simulink model "Combined_Experiment_Jan23_2020a"  (R2020a)
settings: Solver=FixedStepAuto  StartTime=0.0  StopTime=tsim  FixedStep=baseRate  RelTol=1e-3  EnableMultiTasking=on
undefined symbols (not defined in the file): b0, b1, b_out, baseRate, CHASER_ABSOLUTE_POSITION, DiscIntNeverNeededParam, drop_states_ARM, drop_states_BLACK, drop_states_BLUE, drop_states_RED, F_Black_X_nominal, F_Black_Y_nominal, F_Blue_X_nominal, F_Blue_Y_nominal, F_red_X_nominal, F_red_Y_nominal, F_thrusters_BLACK, F_thrusters_BLUE, F_thrusters_RED, Gamma1_el, Gamma1_sh, Gamma1_wr, Gamma2_el, Gamma2_sh, Gamma2_wr, Gamma3_el, Gamma3_sh, Gamma3_wr, Gamma4_el, Gamma4_sh, Gamma4_wr, Gamma5_el, Gamma5_sh, Gamma5_wr, Gamma6_el, Gamma6_sh, Gamma6_wr, home_states_BLACK, home_states_BLUE, home_states_RED, init_states_BLACK, init_states_BLUE, init_states_RED, Kd_tb, Kd_tblue, Kd_tr, Kd_xb, Kd_xblue, Kd_xr, Kd_yb, Kd_yblue, Kd_yr, Kp_tb, Kp_tblue, Kp_tr, Kp_xb, Kp_xblue, Kp_xr, Kp_yb, Kp_yblue ... (+31)
libraries: dspstat3 x18, raspberrypiBasiclib x10, dspsigops x9, embdlinuxlib x8, MainLibrary x8, simulink x7, mspfiltlib x3, dsparch4 x3, etargetslib x1, sensehatlib x1
(part 2 of 11)

== system Combined_Experiment_Jan23_2020a/Manipulator Initialization ==
  Change BLACK Behavior : Subsystem  TreatAsAtomicUnit=on
  Change BLUE Behavior : Subsystem  TreatAsAtomicUnit=on
  Change RED Behavior : Subsystem  TreatAsAtomicUnit=on
  Data Store Read : DataStoreRead  DataStoreName=WhoAmI
  Is this a simulation? : Subsystem
  This IF block determines whether or not to run the BLACK sim/exp : If  NumInputs=2  IfExpression=u1 == 2 & u2 == 0  ShowElse=off
  This IF block determines whether or not to run the BLUE sim/exp : If  NumInputs=2  IfExpression=u1 == 3 & u2 == 0  ShowElse=off
  "This IF block determines whether or not to run the RED sim/exp " : If  NumInputs=2  IfExpression=u1 == 1 & u2 ==0  ShowElse=off
  wires:
  "This IF block determines whether or not to run the RED sim/exp "/1 -> Change RED Behavior/Action
  This IF block determines whether or not to run the BLACK sim/exp/1 -> Change BLACK Behavior/Action
  Is this a simulation?/1(isSim) -> This IF block determines whether or not to run the BLACK sim/exp/2, This IF block determines whether or not to run the BLUE sim/exp/2, "This IF block determines whether or not to run the RED sim/exp "/2
  Data Store Read/1 -> This IF block determines whether or not to run the BLUE sim/exp/1, This IF block determines whether or not to run the BLACK sim/exp/1, "This IF block determines whether or not to run the RED sim/exp "/1
  This IF block determines whether or not to run the BLUE sim/exp/1 -> Change BLUE Behavior/Action

== system Combined_Experiment_Jan23_2020a/Phase #0: Wait for Synchronization ==
  note: In this subsection, the "if" statements are used to determine two things: 1) whether or not a simulation is begin performed,
      | then 2) if an experiment is being performed, then which platform is the diagram compiled on. The "IdentifyPlatform" variable
      | is obtained from a text file location on each platform; each text file contains a unique identifier for each platform.
  Action Port : ActionPort  ActionPortLabel=if(u1 < u2)
  Change BLACK Behavior : Subsystem  TreatAsAtomicUnit=on
  Change BLUE Behavior : Subsystem  TreatAsAtomicUnit=on
  Change RED Behavior : Subsystem  TreatAsAtomicUnit=on
  Data Store Read : DataStoreRead  DataStoreName=WhoAmI
  Is this a simulation? : Subsystem
  This IF block determines whether or not to run the BLACK sim/exp : If  NumInputs=2  IfExpression=u1 == 2 | u2 == 1  ShowElse=off
  This IF block determines whether or not to run the BLUE sim/exp : If  NumInputs=2  IfExpression=u1 == 3 | u2 == 1  ShowElse=off
  "This IF block determines whether or not to run the RED sim/exp " : If  NumInputs=2  IfExpression=u1 == 1 | u2 == 1  ShowElse=off
  wires:
  Is this a simulation?/1(isSim) -> This IF block determines whether or not to run the BLACK sim/exp/2, This IF block determines whether or not to run the BLUE sim/exp/2, "This IF block determines whether or not to run the RED sim/exp "/2
  "This IF block determines whether or not to run the RED sim/exp "/1 -> Change RED Behavior/Action
  This IF block determines whether or not to run the BLACK sim/exp/1 -> Change BLACK Behavior/Action
  Data Store Read/1 -> This IF block determines whether or not to run the BLUE sim/exp/1, This IF block determines whether or not to run the BLACK sim/exp/1, "This IF block determines whether or not to run the RED sim/exp "/1
  This IF block determines whether or not to run the BLUE sim/exp/1 -> Change BLUE Behavior/Action

== system Combined_Experiment_Jan23_2020a/Phase #1: Start Floating  ==
  note: In this subsection, the "if" statements are used to determine two things: 1) whether or not a simulation is begin performed,
      | then 2) if an experiment is being performed, then which platform is the diagram compiled on. The "IdentifyPlatform" variable
      | is obtained from a text file location on each platform; each text file contains a unique identifier for each platform.
  Action Port : ActionPort  ActionPortLabel=elseif(u1 < u3)
  Change BLACK Behavior : Subsystem  TreatAsAtomicUnit=on
  Change BLUE Behavior : Subsystem  TreatAsAtomicUnit=on
  Change RED Behavior : Subsystem  TreatAsAtomicUnit=on
  Data Store Read : DataStoreRead  DataStoreName=WhoAmI
  Is this a simulation? : Subsystem
  This IF block determines whether or not to run the BLACK sim/exp : If  NumInputs=2  IfExpression=u1 == 2 | u2 == 1  ShowElse=off
  This IF block determines whether or not to run the BLUE sim/exp : If  NumInputs=2  IfExpression=u1 == 3 | u2 == 1  ShowElse=off
  "This IF block determines whether or not to run the RED sim/exp " : If  NumInputs=2  IfExpression=u1 == 1 | u2 == 1  ShowElse=off
  wires:
  "This IF block determines whether or not to run the RED sim/exp "/1 -> Change RED Behavior/Action
  This IF block determines whether or not to run the BLACK sim/exp/1 -> Change BLACK Behavior/Action
  Is this a simulation?/1(isSim) -> This IF block determines whether or not to run the BLUE sim/exp/2, This IF block determines whether or not to run the BLACK sim/exp/2, "This IF block determines whether or not to run the RED sim/exp "/2
  This IF block determines whether or not to run the BLUE sim/exp/1 -> Change BLUE Behavior/Action
  Data Store Read/1 -> This IF block determines whether or not to run the BLUE sim/exp/1, This IF block determines whether or not to run the BLACK sim/exp/1, "This IF block determines whether or not to run the RED sim/exp "/1

== system Combined_Experiment_Jan23_2020a/Phase #2: Move to Initial Position ==
  note: In this subsection, the "if" statements are used to determine two things: 1) whether or not a simulation is begin performed,
      | then 2) if an experiment is being performed, then which platform is the diagram compiled on. The "IdentifyPlatform" variable
      | is obtained from a text file location on each platform; each text file contains a unique identifier for each platform.
  Action Port : ActionPort  ActionPortLabel=elseif( u1 < u4)
  Change BLACK Behavior : Subsystem  TreatAsAtomicUnit=on
  Change BLUE Behavior : Subsystem  TreatAsAtomicUnit=on
  Change RED Behavior : Subsystem  TreatAsAtomicUnit=on
  Data Store Read : DataStoreRead  DataStoreName=WhoAmI
  Is this a simulation? : Subsystem
  This IF block determines whether or not to run the BLACK sim/exp : If  NumInputs=2  IfExpression=u1 == 2 | u2 == 1  ShowElse=off
  This IF block determines whether or not to run the BLUE sim/exp : If  NumInputs=2  IfExpression=u1 == 3 | u2 == 1  ShowElse=off
  "This IF block determines whether or not to run the RED sim/exp " : If  NumInputs=2  IfExpression=u1 == 1 | u2 == 1  ShowElse=off
  wires:
  This IF block determines whether or not to run the BLACK sim/exp/1 -> Change BLACK Behavior/Action
  "This IF block determines whether or not to run the RED sim/exp "/1 -> Change RED Behavior/Action
  This IF block determines whether or not to run the BLUE sim/exp/1 -> Change BLUE Behavior/Action
  Is this a simulation?/1(isSim) -> This IF block determines whether or not to run the BLUE sim/exp/2, This IF block determines whether or not to run the BLACK sim/exp/2, "This IF block determines whether or not to run the RED sim/exp "/2
  Data Store Read/1 -> This IF block determines whether or not to run the BLUE sim/exp/1, This IF block determines whether or not to run the BLACK sim/exp/1, "This IF block determines whether or not to run the RED sim/exp "/1

== system Combined_Experiment_Jan23_2020a/Phase #3: Experiment ==
  note: In this subsection, the "if" statements are used to determine two things: 1) whether or not a simulation is begin performed,
      | then 2) if an experiment is being performed, then which platform is the diagram compiled on. The "IdentifyPlatform" variable
      | is obtained from a text file location on each platform; each text file contains a unique identifier for each platform.
  Action Port : ActionPort  ActionPortLabel=elseif( u1 < u5)
  Change BLACK Behavior : Subsystem  TreatAsAtomicUnit=on
  Change BLUE Behavior : Subsystem  TreatAsAtomicUnit=on
  Change RED Behavior : Subsystem  TreatAsAtomicUnit=on
  Data Store Read : DataStoreRead  DataStoreName=WhoAmI
  Is this a simulation? : Subsystem
  This IF block determines whether or not to run the BLACK sim/exp : If  NumInputs=2  IfExpression=u1 == 2 | u2 == 1  ShowElse=off
  This IF block determines whether or not to run the BLUE sim/exp : If  NumInputs=2  IfExpression=u1 == 3 | u2 == 1  ShowElse=off
  "This IF block determines whether or not to run the RED sim/exp " : If  NumInputs=2  IfExpression=u1 == 1 | u2 == 1  ShowElse=off
  wires:
  "This IF block determines whether or not to run the RED sim/exp "/1 -> Change RED Behavior/Action
  This IF block determines whether or not to run the BLACK sim/exp/1 -> Change BLACK Behavior/Action
  Data Store Read/1 -> This IF block determines whether or not to run the BLUE sim/exp/1, This IF block determines whether or not to run the BLACK sim/exp/1, "This IF block determines whether or not to run the RED sim/exp "/1
  Is this a simulation?/1(isSim) -> This IF block determines whether or not to run the BLUE sim/exp/2, This IF block determines whether or not to run the BLACK sim/exp/2, "This IF block determines whether or not to run the RED sim/exp "/2
  This IF block determines whether or not to run the BLUE sim/exp/1 -> Change BLUE Behavior/Action

== system Combined_Experiment_Jan23_2020a/Phase #4: Return Home ==
  note: In this subsection, the "if" statements are used to determine two things: 1) whether or not a simulation is begin performed,
      | then 2) if an experiment is being performed, then which platform is the diagram compiled on. The "IdentifyPlatform" variable
      | is obtained from a text file location on each platform; each text file contains a unique identifier for each platform.
  Action Port : ActionPort  ActionPortLabel=elseif( u1 < u6)
  Change BLACK Behavior : Subsystem  TreatAsAtomicUnit=on
  Change BLUE Behavior : Subsystem  TreatAsAtomicUnit=on
  Change RED Behavior : Subsystem  TreatAsAtomicUnit=on
  Data Store Read : DataStoreRead  DataStoreName=WhoAmI
  Is this a simulation? : Subsystem
  This IF block determines whether or not to run the BLACK sim/exp : If  NumInputs=2  IfExpression=u1 == 2 | u2 == 1  ShowElse=off
  This IF block determines whether or not to run the BLUE sim/exp : If  NumInputs=2  IfExpression=u1 == 3 | u2 == 1  ShowElse=off
  "This IF block determines whether or not to run the RED sim/exp " : If  NumInputs=2  IfExpression=u1 == 1 | u2 == 1  ShowElse=off
  wires:
  "This IF block determines whether or not to run the RED sim/exp "/1 -> Change RED Behavior/Action
  This IF block determines whether or not to run the BLACK sim/exp/1 -> Change BLACK Behavior/Action
  Data Store Read/1 -> This IF block determines whether or not to run the BLUE sim/exp/1, This IF block determines whether or not to run the BLACK sim/exp/1, "This IF block determines whether or not to run the RED sim/exp "/1
  Is this a simulation?/1(isSim) -> This IF block determines whether or not to run the BLUE sim/exp/2, This IF block determines whether or not to run the BLACK sim/exp/2, "This IF block determines whether or not to run the RED sim/exp "/2
  This IF block determines whether or not to run the BLUE sim/exp/1 -> Change BLUE Behavior/Action

== system Combined_Experiment_Jan23_2020a/Phase #5: Hold Home ==
  note: In this subsection, the "if" statements are used to determine two things: 1) whether or not a simulation is begin performed,
      | then 2) if an experiment is being performed, then which platform is the diagram compiled on. The "IdentifyPlatform" variable
      | is obtained from a text file location on each platform; each text file contains a unique identifier for each platform.
  note: To change the behavior of RED during this phase, double click on the "Change RED Behavior". For BLACK, double click on "Change BLACK Behavior"
  Action Port : ActionPort  ActionPortLabel=elseif( u1 < u7 )
  Change BLACK Behavior : Subsystem  TreatAsAtomicUnit=on
  Change BLUE Behavior : Subsystem  TreatAsAtomicUnit=on
  Change RED Behavior : Subsystem  TreatAsAtomicUnit=on
  Data Store Read : DataStoreRead  DataStoreName=WhoAmI
  Is this a simulation? : Subsystem
  This IF block determines whether or not to run the BLACK sim/exp : If  NumInputs=2  IfExpression=u1 == 2 | u2 == 1  ShowElse=off
  This IF block determines whether or not to run the BLUE sim/exp : If  NumInputs=2  IfExpression=u1 == 3 | u2 == 1  ShowElse=off
  "This IF block determines whether or not to run the RED sim/exp " : If  NumInputs=2  IfExpression=u1 == 1 | u2 == 1  ShowElse=off
  wires:
  "This IF block determines whether or not to run the RED sim/exp "/1 -> Change RED Behavior/Action
  This IF block determines whether or not to run the BLACK sim/exp/1 -> Change BLACK Behavior/Action
  Data Store Read/1 -> This IF block determines whether or not to run the BLUE sim/exp/1, This IF block determines whether or not to run the BLACK sim/exp/1, "This IF block determines whether or not to run the RED sim/exp "/1
  This IF block determines whether or not to run the BLUE sim/exp/1 -> Change BLUE Behavior/Action
  Is this a simulation?/1(isSim) -> This IF block determines whether or not to run the BLACK sim/exp/2, This IF block determines whether or not to run the BLUE sim/exp/2, "This IF block determines whether or not to run the RED sim/exp "/2

== system Combined_Experiment_Jan23_2020a/Phase #6: Stop Floating and Spin Down RW ==
  note: In this subsection, the "if" statements are used to determine two things: 1) whether or not a simulation is begin performed,
      | then 2) if an experiment is being performed, then which platform is the diagram compiled on. The "IdentifyPlatform" variable
      | is obtained from a text file location on each platform; each text file contains a unique identifier for each platform.
  Action Port : ActionPort  ActionPortLabel=else
  Change BLACK Behavior : Subsystem  TreatAsAtomicUnit=on
  Change BLUE Behavior : Subsystem  TreatAsAtomicUnit=on
  Change RED Behavior : Subsystem  TreatAsAtomicUnit=on
  Data Store Read : DataStoreRead  DataStoreName=WhoAmI
  Is this a simulation? : Subsystem
  This IF block determines whether or not to run the BLACK sim/exp : If  NumInputs=2  IfExpression=u1 == 2 | u2 == 1  ShowElse=off
  This IF block determines whether or not to run the BLUE sim/exp : If  NumInputs=2  IfExpression=u1 == 3 | u2 == 1  ShowElse=off
  "This IF block determines whether or not to run the RED sim/exp " : If  NumInputs=2  IfExpression=u1 == 1 | u2 == 1  ShowElse=off
  wires:
  "This IF block determines whether or not to run the RED sim/exp "/1 -> Change RED Behavior/Action
  This IF block determines whether or not to run the BLACK sim/exp/1 -> Change BLACK Behavior/Action
  Is this a simulation?/1(isSim) -> This IF block determines whether or not to run the BLUE sim/exp/2, This IF block determines whether or not to run the BLACK sim/exp/2, "This IF block determines whether or not to run the RED sim/exp "/2
  This IF block determines whether or not to run the BLUE sim/exp/1 -> Change BLUE Behavior/Action
  Data Store Read/1 -> This IF block determines whether or not to run the BLACK sim/exp/1, This IF block determines whether or not to run the BLUE sim/exp/1, "This IF block determines whether or not to run the RED sim/exp "/1

== system Combined_Experiment_Jan23_2020a/Platform Identification ==
  Data Store Write : DataStoreWrite  DataStoreName=WhoAmI
  WhoAmI : MainLibrary/PhaseSpace Functions/WhoAmI  SampleTime=0.1
      settings: SourceProductName=SPOT Custom Library
  wires:
  WhoAmI/1 -> Data Store Write/1

== system Combined_Experiment_Jan23_2020a/Simulate Plant Dynamics ==
  Action Port : ActionPort  ActionPortLabel=if(u1 == 1)
  BLACK Dynamics : Subsystem
  BLUE Dynamics : Subsystem
  IMU Model : Subsystem
  RED and ARM Dynamics : Subsystem

== system Combined_Experiment_Jan23_2020a/Subsystem ==
  Universal_Time : DataStoreRead  DataStoreName=Univ_Time
  Time : Outport  VectorParamsAs1DForOutWhenUnconnected=off
  wires:
  Universal_Time/1 -> Time/1

== system Combined_Experiment_Jan23_2020a/Float & Magnet Controls/Change Behavior ==
  Action Port : ActionPort  ActionPortLabel=if(u1 == 0)
  Data Store Read : DataStoreRead  Commented=on  DataStoreName=Magnet_State
  Data Store Read1 : DataStoreRead  DataStoreName=Float_State
  GPIO for Magnet : embdlinuxlib/GPIO Write  Commented=on  board=Pi 3 Model B  gpio=10  direction=Output  blockPlatform=Raspberry Pi
      settings: SourceProductBaseCode=SC_BEAGLEBONE_BLUE,RASPPI
  GPIO for Pucks : embdlinuxlib/GPIO Write  board=Pi 3 Model B  gpio=26  direction=Output  blockPlatform=Raspberry Pi
      settings: SourceProductBaseCode=SC_BEAGLEBONE_BLUE,RASPPI
  wires:
  Data Store Read1/1 -> GPIO for Pucks/1
  Data Store Read/1 -> GPIO for Magnet/1

== system Combined_Experiment_Jan23_2020a/Float & Magnet Controls/Is this a simulation? ==
  Constant : Constant  Value=simMode  SampleTime=-1
  isSim : Outport  VectorParamsAs1DForOutWhenUnconnected=off
  wires:
  Constant/1 -> isSim/1

== system Combined_Experiment_Jan23_2020a/From ARM Torques Command Joints/Change BLACK Behavior ==
  note: BLACK does not currently have the capability to use a RW.
  Action Port : ActionPort  ActionPortLabel=if(u1 == 2 & u2 == 0)

== system Combined_Experiment_Jan23_2020a/From ARM Torques Command Joints/Change BLUE Behavior ==
  note: BLUE does not currently have the capability to use a RW.
  Action Port : ActionPort  ActionPortLabel=if(u1 == 3 & u2 == 0)

== system Combined_Experiment_Jan23_2020a/From ARM Torques Command Joints/Change RED Behavior ==
  Action Port : ActionPort  ActionPortLabel=if(u1 == 1 & u2 == 0)
  Data Store Read : DataStoreRead  DataStoreName=ARM_Desired_Rz_Shoulder
  Data Store Read1 : DataStoreRead  DataStoreName=ARM_Desired_Rz_Elbow
  Data Store Read2 : DataStoreRead  DataStoreName=ARM_Desired_Rz_Wrist
  Elbow Torque Command : DataStoreRead  Commented=on  DataStoreName=RED_Tz_Elbow
  Send Position Commands to Manipulator : MainLibrary/Dynamixel Functions/Send Position Commands to Manipulator
      settings: SourceProductName=SPOT Custom Library
  Send Torque Commands to Manipulator : MainLibrary/Dynamixel Functions/Send Torque Commands to Manipulator  Commented=on
      settings: SourceProductName=SPOT Custom Library
  Shoulder Torque Command : DataStoreRead  Commented=on  DataStoreName=RED_Tz_Shoulder
  Wrist Torque Command : DataStoreRead  Commented=on  DataStoreName=RED_Tz_Wrist
  wires:
  Shoulder Torque Command/1 -> Send Torque Commands to Manipulator/1
  Elbow Torque Command/1 -> Send Torque Commands to Manipulator/2
  Wrist Torque Command/1 -> Send Torque Commands to Manipulator/3
  Data Store Read/1 -> Send Position Commands to Manipulator/1
  Data Store Read1/1 -> Send Position Commands to Manipulator/2
  Data Store Read2/1 -> Send Position Commands to Manipulator/3

== system Combined_Experiment_Jan23_2020a/From ARM Torques Command Joints/Is this a simulation? ==
  Constant : Constant  Value=simMode  SampleTime=-1
  isSim : Outport  VectorParamsAs1DForOutWhenUnconnected=off
  wires:
  Constant/1 -> isSim/1

== system Combined_Experiment_Jan23_2020a/From Force//Torque to PWM Signal/Change BLACK Behavior ==
  note: Calculate the percentage of time each thruster must be on, and send to the PWM blocks.
  note: Using the attitude, rotate the forces into the body frame.
  note: Calculate which thrusters must be turned on and for how long.
  Action Port : ActionPort  ActionPortLabel=if(u1 == 2 | u2 == 1)
  BLACK_Fx : DataStoreRead  DataStoreName=BLACK_Fx
  BLACK_Fy : DataStoreRead  DataStoreName=BLACK_Fy
  BLACK_Rz : DataStoreRead  DataStoreName=BLACK_Rz
  BLACK_Tz : DataStoreRead  DataStoreName=BLACK_Tz
  Calculate Thruster ON/OFF : Subsystem
  Mux : Mux  Inputs=2
  Mux1 : Mux  Inputs=2
  Rotate Forces to Body : Subsystem
  BLACK PWM : Outport  VectorParamsAs1DForOutWhenUnconnected=off
  wires:
  Rotate Forces to Body/1(F_b) -> Mux1/1
  BLACK_Fx/1 -> Mux/1
  Calculate Thruster ON/OFF/1(ThrusterPWM) -> BLACK PWM/1
  BLACK_Rz/1 -> Rotate Forces to Body/2(Rz)
  Mux/1 -> Rotate Forces to Body/1("F_I ")
  BLACK_Tz/1 -> Mux1/2
  Mux1/1 -> Calculate Thruster ON/OFF/1("[Fx_b; Fy_b; Tz]")
  BLACK_Fy/1 -> Mux/2

== system Combined_Experiment_Jan23_2020a/From Force//Torque to PWM Signal/Change BLUE Behavior ==
  note: Calculate the percentage of time each thruster must be on, and send to the PWM blocks.
  note: Using the attitude, rotate the forces into the body frame.
  note: Calculate which thrusters must be turned on and for how long.
  Action Port : ActionPort  ActionPortLabel=if(u1 == 3 | u2 == 1)
  BLUE_Fx : DataStoreRead  DataStoreName=BLUE_Fx
  BLUE_Fy : DataStoreRead  DataStoreName=BLUE_Fy
  BLUE_Rz : DataStoreRead  DataStoreName=BLUE_Rz
  BLUE_Tz : DataStoreRead  DataStoreName=BLUE_Tz
  Calculate Thruster ON/OFF : Subsystem
  Mux : Mux  Inputs=2
  Mux1 : Mux  Inputs=2
  Rotate Forces to Body : Subsystem
  BLUE PWM : Outport  VectorParamsAs1DForOutWhenUnconnected=off
  wires:
  Rotate Forces to Body/1(F_b) -> Mux1/1
  BLUE_Fx/1 -> Mux/1
  Calculate Thruster ON/OFF/1(ThrusterPWM) -> BLUE PWM/1
  BLUE_Rz/1 -> Rotate Forces to Body/2(Rz)
  Mux/1 -> Rotate Forces to Body/1("F_I ")
  BLUE_Tz/1 -> Mux1/2
  Mux1/1 -> Calculate Thruster ON/OFF/1("[Fx_b; Fy_b; Tz]")
  BLUE_Fy/1 -> Mux/2

== system Combined_Experiment_Jan23_2020a/From Force//Torque to PWM Signal/Change RED Behavior ==
  note: Calculate which thrusters must be turned on and for how long.
  note: Using the attitude, rotate the forces into the body frame.
  note: Calculate the percentage of time each thruster must be on, and send to the PWM blocks.
  Action Port : ActionPort  ActionPortLabel=if(u1 == 1 | u2 == 1)
  Calculate Thruster ON/OFF : Subsystem
  Mux : Mux  Inputs=2
  Mux1 : Mux  Inputs=2
  RED_Fx : DataStoreRead  DataStoreName=RED_Fx
  RED_Fy : DataStoreRead  DataStoreName=RED_Fy
  RED_Rz : DataStoreRead  DataStoreName=RED_Rz
  RED_Tz : DataStoreRead  DataStoreName=RED_Tz
  Rotate Forces to Body : Subsystem
  RED PWM : Outport  VectorParamsAs1DForOutWhenUnconnected=off
  wires:
  RED_Tz/1 -> Mux1/2
  Mux/1 -> Rotate Forces to Body/1("F_I ")
  RED_Fy/1 -> Mux/2
  RED_Fx/1 -> Mux/1
  RED_Rz/1 -> Rotate Forces to Body/2(Rz)
  Rotate Forces to Body/1(F_b) -> Mux1/1
  Calculate Thruster ON/OFF/1(ThrusterPWM) -> RED PWM/1
  Mux1/1 -> Calculate Thruster ON/OFF/1("[Fx_b; Fy_b; Tz]")

== system Combined_Experiment_Jan23_2020a/From Force//Torque to PWM Signal/Is this a simulation? ==
  Constant : Constant  Value=simMode  SampleTime=-1
  isSim : Outport  VectorParamsAs1DForOutWhenUnconnected=off
  wires:
  Constant/1 -> isSim/1

== system Combined_Experiment_Jan23_2020a/From Force//Torque to PWM Signal/Send Commands to PWM Blocks ==
  In1 : Inport
  In2 : Inport  Port=2
  In3 : Inport  Port=3
  In4 : Inport  Port=4
  In5 : Inport  Port=5
  In6 : Inport  Port=6
  In7 : Inport  Port=7
  In8 : Inport  Port=8
  In9 : Inport  Port=9
  BLACK T2 : raspberrypiBasiclib/PWM  board=Pi 3 Model B  Pin_=9  Frequency=10  blockPlatform=Raspberry Pi
      settings: SourceProductBaseCode=RASPPI
  RED T1 - BLACK T8 : raspberrypiBasiclib/PWM  board=Pi 3 Model B  Pin_=27  Frequency=10  blockPlatform=Raspberry Pi
      settings: SourceProductBaseCode=RASPPI
  RED T2 - BLACK T3 : raspberrypiBasiclib/PWM  board=Pi 3 Model B  Pin_=19  Frequency=10  blockPlatform=Raspberry Pi
      settings: SourceProductBaseCode=RASPPI
  RED T3 : raspberrypiBasiclib/PWM  board=Pi 3 Model B  Pin_=4  Frequency=10  blockPlatform=Raspberry Pi
      settings: SourceProductBaseCode=RASPPI
  RED T4 - BLACK T5 : raspberrypiBasiclib/PWM  board=Pi 3 Model B  Pin_=22  Frequency=10  blockPlatform=Raspberry Pi
      settings: SourceProductBaseCode=RASPPI
  RED T5 - BLACK T4 : raspberrypiBasiclib/PWM  board=Pi 3 Model B  Pin_=5  Frequency=10  blockPlatform=Raspberry Pi
      settings: SourceProductBaseCode=RASPPI
  RED T6 - BLACK T7 : raspberrypiBasiclib/PWM  board=Pi 3 Model B  Pin_=6  Frequency=10  blockPlatform=Raspberry Pi
      settings: SourceProductBaseCode=RASPPI
  RED T7 - BLACK T6 : raspberrypiBasiclib/PWM  board=Pi 3 Model B  Pin_=13  Frequency=10  blockPlatform=Raspberry Pi
      settings: SourceProductBaseCode=RASPPI
  RED T8 - BLACK T1 : raspberrypiBasiclib/PWM  board=Pi 3 Model B  Pin_=17  Frequency=10  blockPlatform=Raspberry Pi
      settings: SourceProductBaseCode=RASPPI
  wires:
  In4/1 -> RED T4 - BLACK T5/1
  In5/1 -> RED T5 - BLACK T4/1
  In1/1 -> RED T1 - BLACK T8/1
  In8/1 -> RED T8 - BLACK T1/1
  In9/1 -> BLACK T2/1
  In7/1 -> RED T7 - BLACK T6/1
  In6/1 -> RED T6 - BLACK T7/1
  In3/1 -> RED T3/1
  In2/1 -> RED T2 - BLACK T3/1

== system Combined_Experiment_Jan23_2020a/From Torque Command RW/Change BLACK Behavior ==
  note: BLACK does not currently have the capability to use a RW.
  Action Port : ActionPort

== system Combined_Experiment_Jan23_2020a/From Torque Command RW/Change BLUE Behavior ==
  note: BLUE does not currently have the capability to use a RW.
  Action Port : ActionPort

== system Combined_Experiment_Jan23_2020a/From Torque Command RW/Change RED Behavior ==
  note: In this subsection, the commanded torque is converted to an RPM, which is then saturated based on the known limits of the RW
  note: The saturated wheel RPM is then sent to the wheel controller using PWM blocks.
  Action Port : ActionPort
  Calculate Saturated RPM Signal : Subsystem
  RED_Tz_RW : DataStoreRead  DataStoreName=RED_Tz_RW
  RED_Tz_RW_Sat : DataStoreWrite  DataStoreName=RED_Tz_RW_Sat
  Wheel RPM to PWM : Subsystem
  wires:
  Calculate Saturated RPM Signal/2(RPM_Sat) -> RED_Tz_RW_Sat/1
  RED_Tz_RW/1 -> Calculate Saturated RPM Signal/1(Tz)
  Calculate Saturated RPM Signal/1(RPM) -> Wheel RPM to PWM/1(WheelRPM)

== system Combined_Experiment_Jan23_2020a/From Torque Command RW/Is this a simulation? ==
  Constant : Constant  Value=simMode  SampleTime=-1
  isSim : Outport  VectorParamsAs1DForOutWhenUnconnected=off
  wires:
  Constant/1 -> isSim/1

== system Combined_Experiment_Jan23_2020a/Grab PhaseSpace Data via UDP/Initialize Universal Time (Simulation) ==
  Action Port : ActionPort  ActionPortLabel=elseif(u1 == 1)
  Set Universal Time (If this is a simulation) : Clock
  Universal_Time : DataStoreWrite  DataStoreName=Univ_Time
  wires:
  Set Universal Time (If this is a simulation)/1 -> Universal_Time/1

== system Combined_Experiment_Jan23_2020a/Grab PhaseSpace Data via UDP/Is this a simulation?1 ==
  Constant : Constant  Value=simMode  SampleTime=-1
  isSim : Outport  VectorParamsAs1DForOutWhenUnconnected=off
  wires:
  Constant/1 -> isSim/1

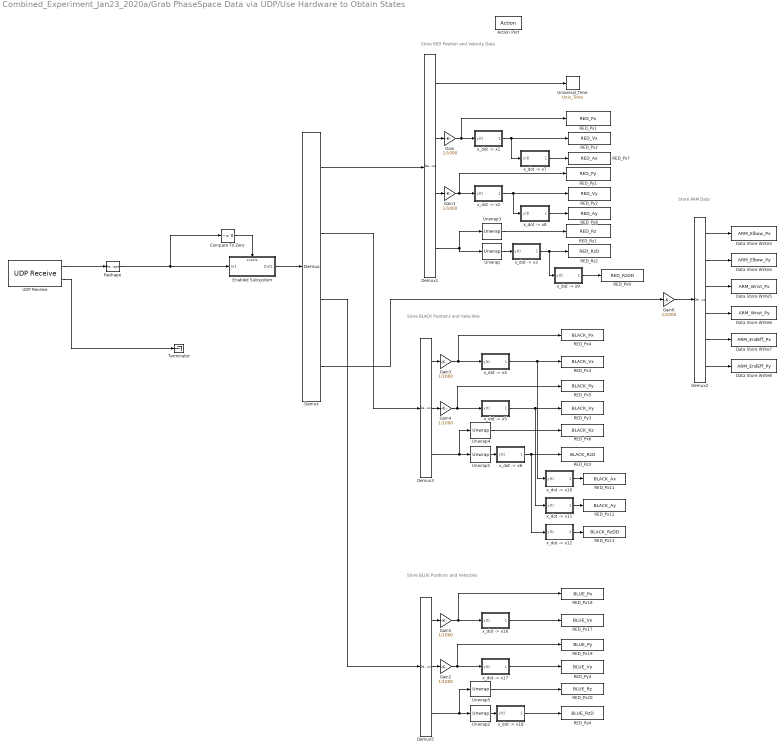
== system Combined_Experiment_Jan23_2020a/Grab PhaseSpace Data via UDP/Use Hardware to Obtain States ==
  note: Store RED Position and Velocity Data
  note: Store ARM Data
  note: Store BLUE Positions and Velocities
  note: Store BLACK Positions and Velocities
  Action Port : ActionPort  ActionPortLabel=if(u1 == 0)
  Compare To Zero : simulink/Logic and Bit Operations/Compare To Zero  relop=~=  OutDataTypeStr=boolean
  Data Store Write3 : DataStoreWrite  DataStoreName=ARM_Elbow_Px
  Data Store Write4 : DataStoreWrite  DataStoreName=ARM_Elbow_Py
  Data Store Write5 : DataStoreWrite  DataStoreName=ARM_Wrist_Px
  Data Store Write6 : DataStoreWrite  DataStoreName=ARM_Wrist_Py
  Data Store Write7 : DataStoreWrite  DataStoreName=ARM_EndEff_Px
  Data Store Write8 : DataStoreWrite  DataStoreName=ARM_EndEff_Py
  Demux : Demux  Outputs=[4,3,3,6]
  Demux1 : Demux
  Demux2 : Demux  Outputs=6
  Demux3 : Demux  Outputs=3
  Demux5 : Demux  Outputs=3
  Enabled Subsystem : Subsystem  TreatAsAtomicUnit=on
  Gain{,1..6} (7 alike) : Gain  Gain=1/1000
  RED_Px1 : DataStoreWrite  DataStoreName=RED_Px
  RED_Px11 : DataStoreWrite  DataStoreName=BLACK_Ax
  RED_Px12 : DataStoreWrite  DataStoreName=BLACK_Ay
  RED_Px13 : DataStoreWrite  DataStoreName=BLACK_RzDD
  RED_Px17 : DataStoreWrite  DataStoreName=BLUE_Vx
  RED_Px18 : DataStoreWrite  DataStoreName=BLUE_Px
  RED_Px19 : DataStoreWrite  DataStoreName=BLUE_Py
  RED_Px2 : DataStoreWrite  DataStoreName=RED_Vx
  RED_Px20 : DataStoreWrite  DataStoreName=BLUE_Rz
  RED_Px3 : DataStoreWrite  DataStoreName=BLACK_Vx
  RED_Px4 : DataStoreWrite  DataStoreName=BLACK_Px
  RED_Px5 : DataStoreWrite  DataStoreName=BLACK_Py
  RED_Px6 : DataStoreWrite  DataStoreName=BLACK_Rz
  RED_Px7 : DataStoreWrite  DataStoreName=RED_Ax
  RED_Px8 : DataStoreWrite  DataStoreName=RED_Ay
  RED_Px9 : DataStoreWrite  DataStoreName=RED_RzDD
  RED_Py1 : DataStoreWrite  DataStoreName=RED_Py
  RED_Py2 : DataStoreWrite  DataStoreName=RED_Vy
  RED_Py3 : DataStoreWrite  DataStoreName=BLACK_Vy
  RED_Py4 : DataStoreWrite  DataStoreName=BLUE_Vy
  RED_Rz1 : DataStoreWrite  DataStoreName=RED_Rz
  RED_Rz2 : DataStoreWrite  DataStoreName=RED_RzD
  RED_Rz3 : DataStoreWrite  DataStoreName=BLACK_RzD
  RED_Rz4 : DataStoreWrite  DataStoreName=BLUE_RzD
  Reshape : Reshape  OutputDimensionality=Customize  OutputDimensions=[16,1]
  Terminator : Terminator
  UDP Receive : embdlinuxlib/UDP Receive  localURL='0.0.0.0'  localPort=31534  remoteURL='0.0.0.0'  remotePort=-1  recvBufferSize=8192  signalDatatype=double  dims=16  isVarSize=off  showBlockingTime=off  blockingTime=0  sampletime=0  blockPlatform=Raspberry Pi
      settings: SourceProductBaseCode=SC_BEAGLEBONE_BLUE,RASPPI
  Universal_Time : DataStoreWrite  DataStoreName=Univ_Time
  Unwrap{,1..5} (6 alike) : dspsigops/Unwrap  tol=pi  InputProcessing=Columns as channels (frame based)  running=off
  "x_dot -> x1" : Subsystem
  "x_dot -> x10" : Subsystem
  "x_dot -> x11" : Subsystem
  "x_dot -> x12" : Subsystem
  "x_dot -> x16" : Subsystem
  "x_dot -> x17" : Subsystem
  "x_dot -> x18" : Subsystem
  "x_dot -> x2" : Subsystem
  "x_dot -> x3" : Subsystem
  "x_dot -> x4" : Subsystem
  "x_dot -> x5" : Subsystem
  "x_dot -> x6" : Subsystem
  "x_dot -> x7" : Subsystem
  "x_dot -> x8" : Subsystem
  "x_dot -> x9" : Subsystem
  wires:
  "x_dot -> x12"/1(dy(t)/dt) -> RED_Px13/1
  "x_dot -> x6"/1(dy(t)/dt) -> RED_Rz3/1, "x_dot -> x12"/1(y(t))
  "x_dot -> x16"/1(dy(t)/dt) -> RED_Px17/1
  Unwrap2/1 -> "x_dot -> x18"/1(y(t))
  Demux3/3 -> Unwrap1/1, Unwrap4/1
  Demux3/2 -> Gain4/1
  Demux5/2 -> Gain2/1
  Demux2/1 -> Data Store Write3/1
  "x_dot -> x1"/1(dy(t)/dt) -> "x_dot -> x7"/1(y(t)), RED_Px2/1
  Demux5/3 -> Unwrap2/1, Unwrap5/1
  Demux5/1 -> Gain5/1
  "x_dot -> x2"/1(dy(t)/dt) -> "x_dot -> x8"/1(y(t)), RED_Py2/1
  "x_dot -> x17"/1(dy(t)/dt) -> RED_Py4/1
  Demux1/3 -> Gain1/1
  Demux2/2 -> Data Store Write4/1
  "x_dot -> x18"/1(dy(t)/dt) -> RED_Rz4/1
  Demux/1 -> Demux1/1
  "x_dot -> x8"/1(dy(t)/dt) -> RED_Px8/1
  Unwrap/1 -> "x_dot -> x3"/1(y(t))
  Demux/2 -> Demux3/1
  Demux2/6 -> Data Store Write8/1
  Demux2/5 -> Data Store Write7/1
  "x_dot -> x10"/1(dy(t)/dt) -> RED_Px11/1
  "x_dot -> x3"/1(dy(t)/dt) -> "x_dot -> x9"/1(y(t)), RED_Rz2/1
  "x_dot -> x7"/1(dy(t)/dt) -> RED_Px7/1
  "x_dot -> x11"/1(dy(t)/dt) -> RED_Px12/1
  "x_dot -> x5"/1(dy(t)/dt) -> RED_Py3/1, "x_dot -> x11"/1(y(t))
  Unwrap1/1 -> "x_dot -> x6"/1(y(t))
  "x_dot -> x4"/1(dy(t)/dt) -> "x_dot -> x10"/1(y(t)), RED_Px3/1
  Demux3/1 -> Gain3/1
  Demux2/4 -> Data Store Write6/1
  Demux1/2 -> Gain/1
  Demux2/3 -> Data Store Write5/1
  "x_dot -> x9"/1(dy(t)/dt) -> RED_Px9/1
  UDP Receive/1 -> Reshape/1
  Reshape/1 -> Enabled Subsystem/1(In1), Compare To Zero/1
  Compare To Zero/1 -> Enabled Subsystem/Enable
  Enabled Subsystem/1(Out1) -> Demux/1
  Demux1/1 -> Universal_Time/1
  UDP Receive/2 -> Terminator/1
  Demux/4 -> Gain6/1
  Demux/3 -> Demux5/1
  Gain/1 -> "x_dot -> x1"/1(y(t)), RED_Px1/1
  Gain1/1 -> "x_dot -> x2"/1(y(t)), RED_Py1/1
  Demux1/4 -> Unwrap/1, Unwrap3/1
  Gain3/1 -> "x_dot -> x4"/1(y(t)), RED_Px4/1
  Gain4/1 -> "x_dot -> x5"/1(y(t)), RED_Px5/1
  Gain5/1 -> "x_dot -> x16"/1(y(t)), RED_Px18/1
  Gain2/1 -> "x_dot -> x17"/1(y(t)), RED_Px19/1
  Gain6/1 -> Demux2/1
  Unwrap3/1 -> RED_Rz1/1
  Unwrap4/1 -> RED_Px6/1
  Unwrap5/1 -> RED_Px20/1

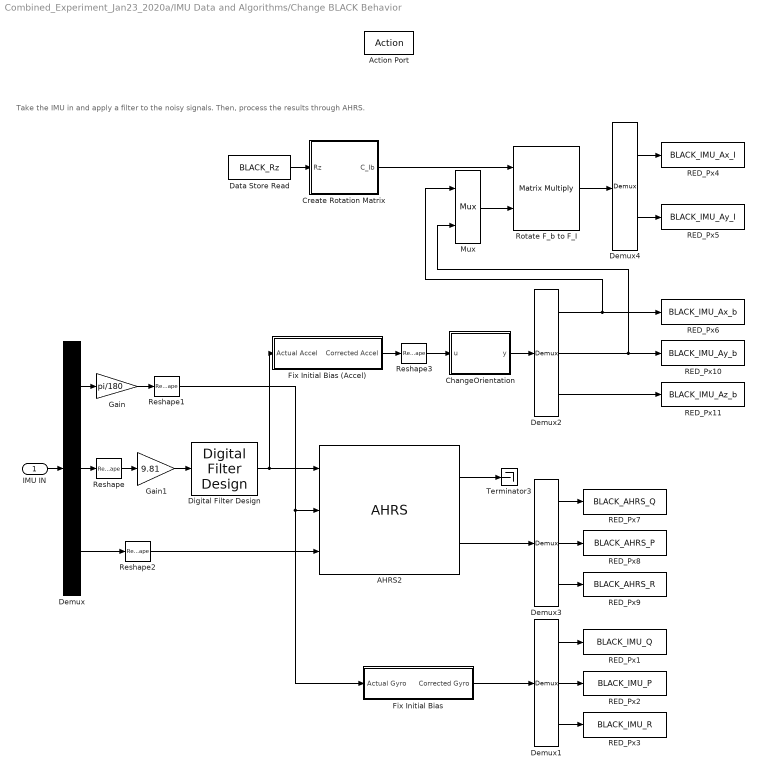
== system Combined_Experiment_Jan23_2020a/IMU Data and Algorithms/Change BLACK Behavior ==
  note: Take the IMU in and apply a filter to the noisy signals. Then, process the results through AHRS.
  IMU IN : Inport
  Action Port : ActionPort  ActionPortLabel=if(u1 == 2 & u2 == 0)
  AHRS2 : mspfiltlib/AHRS  DispRefFrame=NED  DecimationFactor=1  InitialProcessNoise=ahrsfilter.defaultProcessNoise  OrientationFormat=quaternion  SimulateUsing=Interpreted execution  AccelerometerNoise=0.0001924722  GyroscopeNoise=9.1385e-5  MagnetometerNoise=0.1  GyroscopeDriftNoise=3.0462e-13  LinearAccelerationNoise=0.0096236100000000012  MagneticDisturbanceNoise=0.5  LinearAccelerationDecayFactor=0.5  MagneticDisturbanceDecayFactor=0.5  ExpectedMagneticFieldStrength=33
      settings: SourceProductBaseCode=TF,NV
  ChangeOrientation : MATLAB Function  TreatAsAtomicUnit=on
  Create Rotation Matrix : MATLAB Function  TreatAsAtomicUnit=on
  Data Store Read : DataStoreRead  DataStoreName=BLACK_Rz
  Demux : Demux  Outputs=[3,3,3]
  Demux1 : Demux  Outputs=3
  Demux2 : Demux  Outputs=3
  Demux3 : Demux  Outputs=3
  Demux4 : Demux  Outputs=2
  Digital Filter Design : dsparch4/Digital Filter Design  mwdsp_browser_bugfix_var=off
  Fix Initial Bias : Subsystem
  Fix Initial Bias (Accel) : Subsystem
  Gain : Gain  Gain=pi/180
  Gain1 : Gain  Gain=9.81
  Mux : Mux  Inputs=2
  RED_Px1 : DataStoreWrite  DataStoreName=BLACK_IMU_Q
  RED_Px10 : DataStoreWrite  DataStoreName=BLACK_IMU_Ay_b
  RED_Px11 : DataStoreWrite  DataStoreName=BLACK_IMU_Az_b
  RED_Px2 : DataStoreWrite  DataStoreName=BLACK_IMU_P
  RED_Px3 : DataStoreWrite  DataStoreName=BLACK_IMU_R
  RED_Px4 : DataStoreWrite  DataStoreName=BLACK_IMU_Ax_I
  RED_Px5 : DataStoreWrite  DataStoreName=BLACK_IMU_Ay_I
  RED_Px6 : DataStoreWrite  DataStoreName=BLACK_IMU_Ax_b
  RED_Px7 : DataStoreWrite  DataStoreName=BLACK_AHRS_Q
  RED_Px8 : DataStoreWrite  DataStoreName=BLACK_AHRS_P
  RED_Px9 : DataStoreWrite  DataStoreName=BLACK_AHRS_R
  Reshape{,1..3} (4 alike) : Reshape  OutputDimensionality=Row vector (2-D)
  Rotate F_b to F_I : Product  Multiplication=Matrix(*)
  Terminator3 : Terminator
  wires:
  Demux3/2 -> RED_Px8/1
  Reshape/1 -> Gain1/1
  Demux3/1 -> RED_Px7/1
  AHRS2/1 -> Terminator3/1
  AHRS2/2 -> Demux3/1
  Demux3/3 -> RED_Px9/1
  Gain/1 -> Reshape1/1
  Demux2/3 -> RED_Px11/1
  Reshape2/1 -> AHRS2/3
  Demux/1 -> Gain/1
  Demux/2 -> Reshape/1
  IMU IN/1 -> Demux/1
  Demux/3 -> Reshape2/1
  Demux1/2 -> RED_Px2/1
  Fix Initial Bias/1(Corrected Gyro) -> Demux1/1
  Demux1/1 -> RED_Px1/1
  Fix Initial Bias (Accel)/1(Corrected Accel) -> Reshape3/1
  Demux1/3 -> RED_Px3/1
  ChangeOrientation/1(y) -> Demux2/1
  Gain1/1 -> Digital Filter Design/1
  Reshape3/1 -> ChangeOrientation/1(u)
  Digital Filter Design/1 -> Fix Initial Bias (Accel)/1(Actual Accel), AHRS2/1
  Reshape1/1 -> Fix Initial Bias/1(Actual Gyro), AHRS2/2
  Create Rotation Matrix/1(C_Ib) -> Rotate F_b to F_I/1
  Rotate F_b to F_I/1 -> Demux4/1
  Mux/1 -> Rotate F_b to F_I/2
  Data Store Read/1 -> Create Rotation Matrix/1(Rz)
  Demux4/1 -> RED_Px4/1
  Demux2/2 -> Mux/2, RED_Px10/1
  Demux2/1 -> Mux/1, RED_Px6/1
  Demux4/2 -> RED_Px5/1

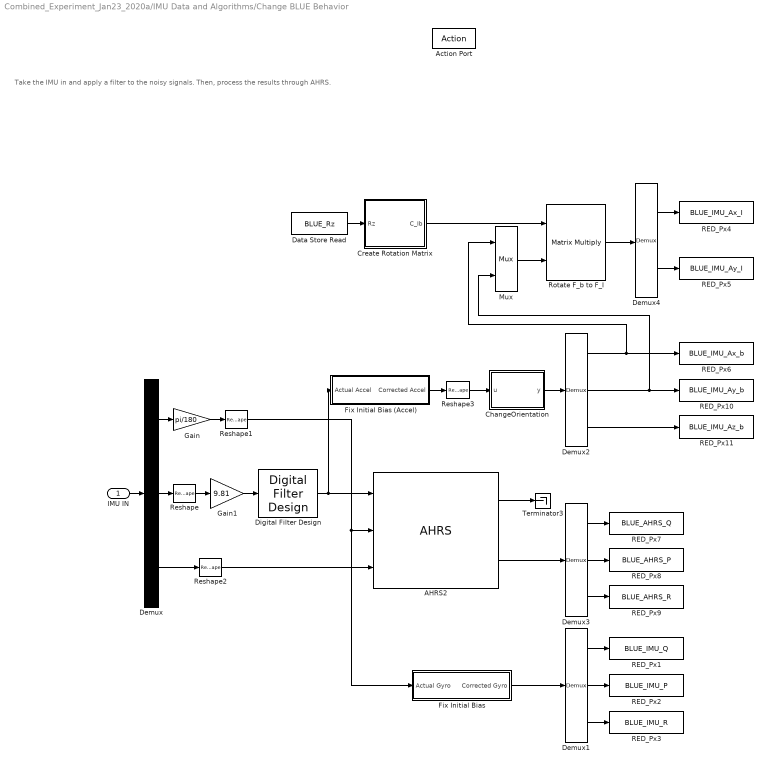
== system Combined_Experiment_Jan23_2020a/IMU Data and Algorithms/Change BLUE Behavior ==
  note: Take the IMU in and apply a filter to the noisy signals. Then, process the results through AHRS.
  IMU IN : Inport
  Action Port : ActionPort  ActionPortLabel=if(u1 == 3 & u2 == 0)
  AHRS2 : mspfiltlib/AHRS  DispRefFrame=NED  DecimationFactor=1  InitialProcessNoise=ahrsfilter.defaultProcessNoise  OrientationFormat=quaternion  SimulateUsing=Interpreted execution  AccelerometerNoise=0.0001924722  GyroscopeNoise=9.1385e-5  MagnetometerNoise=0.1  GyroscopeDriftNoise=3.0462e-13  LinearAccelerationNoise=0.0096236100000000012  MagneticDisturbanceNoise=0.5  LinearAccelerationDecayFactor=0.5  MagneticDisturbanceDecayFactor=0.5  ExpectedMagneticFieldStrength=33
      settings: SourceProductBaseCode=TF,NV
  ChangeOrientation : MATLAB Function  TreatAsAtomicUnit=on
  Create Rotation Matrix : MATLAB Function  TreatAsAtomicUnit=on
  Data Store Read : DataStoreRead  DataStoreName=BLUE_Rz
  Demux : Demux  Outputs=[3,3,3]
  Demux1 : Demux  Outputs=3
  Demux2 : Demux  Outputs=3
  Demux3 : Demux  Outputs=3
  Demux4 : Demux  Outputs=2
  Digital Filter Design : dsparch4/Digital Filter Design  mwdsp_browser_bugfix_var=off
  Fix Initial Bias : Subsystem
  Fix Initial Bias (Accel) : Subsystem
  Gain : Gain  Gain=pi/180
  Gain1 : Gain  Gain=9.81
  Mux : Mux  Inputs=2
  RED_Px1 : DataStoreWrite  DataStoreName=BLUE_IMU_Q
  RED_Px10 : DataStoreWrite  DataStoreName=BLUE_IMU_Ay_b
  RED_Px11 : DataStoreWrite  DataStoreName=BLUE_IMU_Az_b
  RED_Px2 : DataStoreWrite  DataStoreName=BLUE_IMU_P
  RED_Px3 : DataStoreWrite  DataStoreName=BLUE_IMU_R
  RED_Px4 : DataStoreWrite  DataStoreName=BLUE_IMU_Ax_I
  RED_Px5 : DataStoreWrite  DataStoreName=BLUE_IMU_Ay_I
  RED_Px6 : DataStoreWrite  DataStoreName=BLUE_IMU_Ax_b
  RED_Px7 : DataStoreWrite  DataStoreName=BLUE_AHRS_Q
  RED_Px8 : DataStoreWrite  DataStoreName=BLUE_AHRS_P
  RED_Px9 : DataStoreWrite  DataStoreName=BLUE_AHRS_R
  Reshape{,1..3} (4 alike) : Reshape  OutputDimensionality=Row vector (2-D)
  Rotate F_b to F_I : Product  Multiplication=Matrix(*)
  Terminator3 : Terminator
  wires:
  Demux/2 -> Reshape/1
  Demux1/1 -> RED_Px1/1
  Gain1/1 -> Digital Filter Design/1
  Fix Initial Bias (Accel)/1(Corrected Accel) -> Reshape3/1
  Demux1/3 -> RED_Px3/1
  Reshape/1 -> Gain1/1
  Fix Initial Bias/1(Corrected Gyro) -> Demux1/1
  Reshape3/1 -> ChangeOrientation/1(u)
  Demux1/2 -> RED_Px2/1
  Demux/3 -> Reshape2/1
  IMU IN/1 -> Demux/1
  Reshape2/1 -> AHRS2/3
  Gain/1 -> Reshape1/1
  Demux3/2 -> RED_Px8/1
  AHRS2/1 -> Terminator3/1
  Demux3/1 -> RED_Px7/1
  Digital Filter Design/1 -> Fix Initial Bias (Accel)/1(Actual Accel), AHRS2/1
  Reshape1/1 -> Fix Initial Bias/1(Actual Gyro), AHRS2/2
  Rotate F_b to F_I/1 -> Demux4/1
  Mux/1 -> Rotate F_b to F_I/2
  Demux4/1 -> RED_Px4/1
  ChangeOrientation/1(y) -> Demux2/1
  Demux/1 -> Gain/1
  Demux2/1 -> Mux/1, RED_Px6/1
  Data Store Read/1 -> Create Rotation Matrix/1(Rz)
  Demux2/2 -> Mux/2, RED_Px10/1
  Demux2/3 -> RED_Px11/1
  Demux4/2 -> RED_Px5/1
  Demux3/3 -> RED_Px9/1
  AHRS2/2 -> Demux3/1
  Create Rotation Matrix/1(C_Ib) -> Rotate F_b to F_I/1

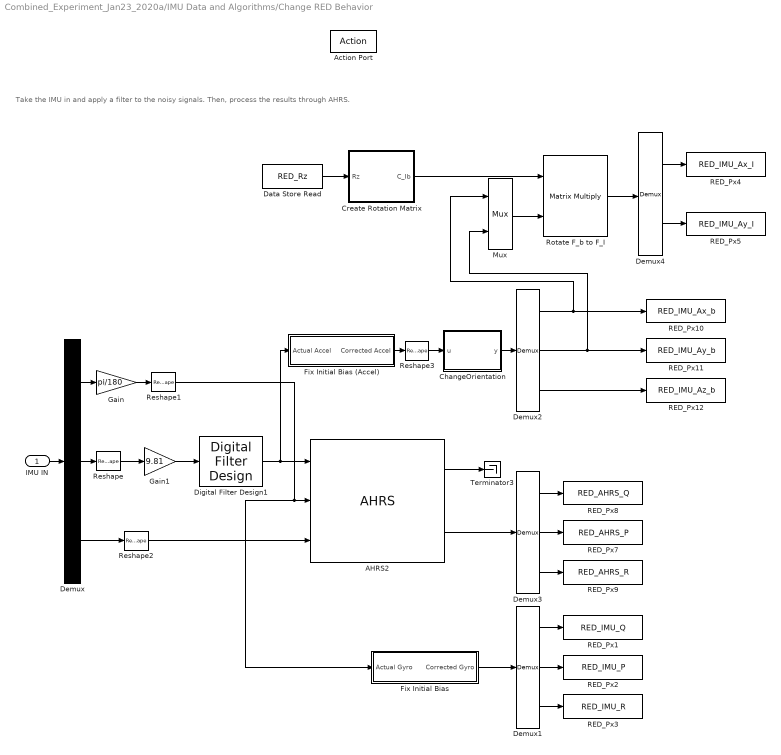
== system Combined_Experiment_Jan23_2020a/IMU Data and Algorithms/Change RED Behavior ==
  note: Take the IMU in and apply a filter to the noisy signals. Then, process the results through AHRS.
  IMU IN : Inport
  Action Port : ActionPort  ActionPortLabel=if(u1 == 1 & u2 ==0)
  AHRS2 : mspfiltlib/AHRS  DispRefFrame=NED  DecimationFactor=1  InitialProcessNoise=ahrsfilter.defaultProcessNoise  OrientationFormat=quaternion  SimulateUsing=Interpreted execution  AccelerometerNoise=0.0001924722  GyroscopeNoise=9.1385e-5  MagnetometerNoise=0.1  GyroscopeDriftNoise=3.0462e-13  LinearAccelerationNoise=0.0096236100000000012  MagneticDisturbanceNoise=0.5  LinearAccelerationDecayFactor=0.5  MagneticDisturbanceDecayFactor=0.5  ExpectedMagneticFieldStrength=33
      settings: SourceProductBaseCode=TF,NV
  ChangeOrientation : MATLAB Function  TreatAsAtomicUnit=on
  Create Rotation Matrix : MATLAB Function  TreatAsAtomicUnit=on
  Data Store Read : DataStoreRead  DataStoreName=RED_Rz
  Demux : Demux  Outputs=[3,3,3]
  Demux1 : Demux  Outputs=3
  Demux2 : Demux  Outputs=3
  Demux3 : Demux  Outputs=3
  Demux4 : Demux  Outputs=2
  Digital Filter Design1 : dsparch4/Digital Filter Design  mwdsp_browser_bugfix_var=off
  Fix Initial Bias : Subsystem
  Fix Initial Bias (Accel) : Subsystem
  Gain : Gain  Gain=pi/180
  Gain1 : Gain  Gain=9.81
  Mux : Mux  Inputs=2
  RED_Px1 : DataStoreWrite  DataStoreName=RED_IMU_Q
  RED_Px10 : DataStoreWrite  DataStoreName=RED_IMU_Ax_b
  RED_Px11 : DataStoreWrite  DataStoreName=RED_IMU_Ay_b
  RED_Px12 : DataStoreWrite  DataStoreName=RED_IMU_Az_b
  RED_Px2 : DataStoreWrite  DataStoreName=RED_IMU_P
  RED_Px3 : DataStoreWrite  DataStoreName=RED_IMU_R
  RED_Px4 : DataStoreWrite  DataStoreName=RED_IMU_Ax_I
  RED_Px5 : DataStoreWrite  DataStoreName=RED_IMU_Ay_I
  RED_Px7 : DataStoreWrite  DataStoreName=RED_AHRS_P
  RED_Px8 : DataStoreWrite  DataStoreName=RED_AHRS_Q
  RED_Px9 : DataStoreWrite  DataStoreName=RED_AHRS_R
  Reshape{,1..3} (4 alike) : Reshape  OutputDimensionality=Row vector (2-D)
  Rotate F_b to F_I : Product  Multiplication=Matrix(*)
  Terminator3 : Terminator
  wires:
  Reshape2/1 -> AHRS2/3
  Gain/1 -> Reshape1/1
  Demux2/3 -> RED_Px12/1
  Demux3/3 -> RED_Px9/1
  AHRS2/2 -> Demux3/1
  AHRS2/1 -> Terminator3/1
  Reshape/1 -> Gain1/1
  Demux/2 -> Reshape/1
  Demux/3 -> Reshape2/1
  Demux/1 -> Gain/1
  IMU IN/1 -> Demux/1
  Demux1/1 -> RED_Px1/1
  Demux1/2 -> RED_Px2/1
  Demux1/3 -> RED_Px3/1
  Fix Initial Bias/1(Corrected Gyro) -> Demux1/1
  ChangeOrientation/1(y) -> Demux2/1
  Demux3/2 -> RED_Px7/1
  Demux3/1 -> RED_Px8/1
  Digital Filter Design1/1 -> Fix Initial Bias (Accel)/1(Actual Accel), AHRS2/1
  Gain1/1 -> Digital Filter Design1/1
  Reshape3/1 -> ChangeOrientation/1(u)
  Fix Initial Bias (Accel)/1(Corrected Accel) -> Reshape3/1
  Reshape1/1 -> Fix Initial Bias/1(Actual Gyro), AHRS2/2
  Data Store Read/1 -> Create Rotation Matrix/1(Rz)
  Mux/1 -> Rotate F_b to F_I/2
  Rotate F_b to F_I/1 -> Demux4/1
  Create Rotation Matrix/1(C_Ib) -> Rotate F_b to F_I/1
  Demux2/2 -> Mux/2, RED_Px11/1
  Demux4/1 -> RED_Px4/1
  Demux4/2 -> RED_Px5/1
  Demux2/1 -> Mux/1, RED_Px10/1

== system Combined_Experiment_Jan23_2020a/IMU Data and Algorithms/Is this a simulation? ==
  Constant : Constant  Value=simMode  SampleTime=-1
  isSim : Outport  VectorParamsAs1DForOutWhenUnconnected=off
  wires:
  Constant/1 -> isSim/1

== system Combined_Experiment_Jan23_2020a/Jetson Communication/Kirk Network Control (EXP) ==
  Action Port : ActionPort  ActionPortLabel=if((u1 == 1 & u2 == 0) & (u3 > u4) & (u3 < u5) )
  " " : DataStoreRead  DataStoreName=Univ_Time
  Add : Sum  Inputs=+-
  Constant : Constant  Value=1.00
  Constant5 : Constant  Value=Phase2_End
  Data Store Read10 : DataStoreRead  DataStoreName=BLACK_Vy
  Data Store Read11 : DataStoreRead  DataStoreName=BLACK_RzD
  Data Store Read12 : DataStoreRead  DataStoreName=ZED_ProcessingTime
  Data Store Read13 : DataStoreRead  DataStoreName=ZED_Confidence
  Data Store Read14 : DataStoreRead  DataStoreName=ZED_Yaw
  Data Store Read15 : DataStoreRead  DataStoreName=ZED_Relative_Y
  Data Store Read16 : DataStoreRead  DataStoreName=ZED_Relative_X
  Data Store Read17 : DataStoreRead  DataStoreName=BLACK_Py
  Data Store Read18 : DataStoreRead  DataStoreName=BLACK_Rz
  Data Store Read19 : DataStoreRead  DataStoreName=BLACK_Px
  Data Store Read22 : DataStoreRead  DataStoreName=BLACK_Vx
  Data Store Read4 : DataStoreRead  DataStoreName=RED_Px
  Data Store Read5 : DataStoreRead  DataStoreName=RED_Py
  Data Store Read6 : DataStoreRead  DataStoreName=RED_Rz
  Data Store Read7 : DataStoreRead  DataStoreName=RED_Vx
  Data Store Read8 : DataStoreRead  DataStoreName=RED_Vy
  Data Store Read9 : DataStoreRead  DataStoreName=RED_RzD
  Data Store Write4 : DataStoreWrite  DataStoreName=RED_Desired_Ax
  Data Store Write5 : DataStoreWrite  DataStoreName=RED_Desired_Ay
  Data Store Write6 : DataStoreWrite  DataStoreName=RED_Desired_Alpha
  MATLAB Function : MATLAB Function  TreatAsAtomicUnit=on
  wires:
  Data Store Read11/1 -> MATLAB Function/13(Pi_black_omega)
  Data Store Read7/1 -> MATLAB Function/5(Pi_red_Vx)
  " "/1 -> Add/1
  Data Store Read18/1 -> MATLAB Function/10(Pi_black_theta)
  Data Store Read17/1 -> MATLAB Function/9(Pi_black_y)
  Data Store Read8/1 -> MATLAB Function/6(Pi_red_Vy)
  MATLAB Function/2(Ay_command) -> Data Store Write5/1
  Data Store Read10/1 -> MATLAB Function/12(Pi_black_Vy)
  Data Store Read22/1 -> MATLAB Function/11(Pi_black_Vx)
  Data Store Read19/1 -> MATLAB Function/8(Pi_black_x)
  Data Store Read5/1 -> MATLAB Function/3(Pi_red_y)
  Add/1 -> MATLAB Function/1(Pi_time)
  Data Store Read9/1 -> MATLAB Function/7(Pi_red_omega)
  Constant5/1 -> Add/2
  Data Store Read15/1 -> MATLAB Function/16(ZED_Relative_Y)
  Data Store Read13/1 -> MATLAB Function/18(ZED_Confidence)
  MATLAB Function/3(Az_command) -> Data Store Write6/1
  Data Store Read12/1 -> MATLAB Function/14(ZED_Processing_Time)
  MATLAB Function/1(Ax_command) -> Data Store Write4/1
  Data Store Read6/1 -> MATLAB Function/4(Pi_red_theta)
  Data Store Read4/1 -> MATLAB Function/2(Pi_red_x)
  Data Store Read16/1 -> MATLAB Function/15(ZED_Relative_X)
  Data Store Read14/1 -> MATLAB Function/17(ZED_Yaw)
  Constant/1 -> MATLAB Function/19(HOLD_POINT_RADIUS)

== system Combined_Experiment_Jan23_2020a/Jetson Communication/Kirk Network Control (SIM) ==
  Action Port : ActionPort  ActionPortLabel=elseif((u2 == 1) & (u3 > u4) & (u3 < u5) )
  " " : DataStoreRead  DataStoreName=Univ_Time
  Add : Sum  Inputs=+-
  Constant : Constant  Value=1.00
  Constant5 : Constant  Value=Phase2_End
  Data Store Read : DataStoreRead  DataStoreName=RED_Px
  Data Store Read1 : DataStoreRead  DataStoreName=RED_Py
  Data Store Read10 : DataStoreRead  DataStoreName=BLACK_Vy
  Data Store Read11 : DataStoreRead  DataStoreName=BLACK_RzD
  Data Store Read17 : DataStoreRead  DataStoreName=BLACK_Py
  Data Store Read18 : DataStoreRead  DataStoreName=BLACK_Rz
  Data Store Read2 : DataStoreRead  DataStoreName=RED_Rz
  Data Store Read22 : DataStoreRead  DataStoreName=BLACK_Vx
  Data Store Read6 : DataStoreRead  DataStoreName=RED_Vx
  Data Store Read7 : DataStoreRead  DataStoreName=RED_Vy
  Data Store Read8 : DataStoreRead  DataStoreName=RED_RzD
  Data Store Read9 : DataStoreRead  DataStoreName=BLACK_Px
  Data Store Write3 : DataStoreWrite  DataStoreName=RED_Desired_Ax
  Data Store Write4 : DataStoreWrite  DataStoreName=RED_Desired_Ay
  Data Store Write5 : DataStoreWrite  DataStoreName=RED_Desired_Alpha
  MATLAB Function : MATLAB Function  TreatAsAtomicUnit=on
  Zero-Order Hold : ZeroOrderHold  SampleTime=0.5
  Zero-Order Hold1 : ZeroOrderHold  SampleTime=0.5
  Zero-Order Hold2 : ZeroOrderHold  SampleTime=0.5
  wires:
  Data Store Read1/1 -> MATLAB Function/3(Pi_red_y)
  Data Store Read/1 -> MATLAB Function/2(Pi_red_x)
  Data Store Read2/1 -> MATLAB Function/4(Pi_red_theta)
  Data Store Read9/1 -> Zero-Order Hold/1
  Data Store Read17/1 -> Zero-Order Hold1/1
  Data Store Read18/1 -> Zero-Order Hold2/1
  MATLAB Function/1(Ax_command) -> Data Store Write3/1
  MATLAB Function/2(Ay_command) -> Data Store Write4/1
  MATLAB Function/3(Az_command) -> Data Store Write5/1
  Data Store Read6/1 -> MATLAB Function/5(Pi_red_Vx)
  Data Store Read7/1 -> MATLAB Function/6(Pi_red_Vy)
  Data Store Read8/1 -> MATLAB Function/7(Pi_red_omega)
  Data Store Read22/1 -> MATLAB Function/11(Pi_black_Vx)
  Data Store Read10/1 -> MATLAB Function/12(Pi_black_Vy)
  Data Store Read11/1 -> MATLAB Function/13(Pi_black_omega)
  " "/1 -> Add/1
  Add/1 -> MATLAB Function/1(Pi_time)
  Constant5/1 -> Add/2
  Zero-Order Hold/1 -> MATLAB Function/8(Pi_black_x)
  Zero-Order Hold1/1 -> MATLAB Function/9(Pi_black_y)
  Zero-Order Hold2/1 -> MATLAB Function/10(Pi_black_theta)
  Constant/1 -> MATLAB Function/14(HOLD_POINT_RADIUS)

== system Combined_Experiment_Jan23_2020a/Jetson Communication/isSim ==
  Constant : Constant  Value=simMode  SampleTime=-1
  isSim : Outport  VectorParamsAs1DForOutWhenUnconnected=off
  wires:
  Constant/1 -> isSim/1

== system Combined_Experiment_Jan23_2020a/Manipulator Encoder Data/Change Behavior ==
  Action Port : ActionPort  ActionPortLabel=if(u1 == 0)
  Correct for dropouts : Subsystem
  Correct for dropouts1 : Subsystem
  Correct for dropouts2 : Subsystem
  Data Store Write : DataStoreWrite  DataStoreName=RED_Rz_Shoulder
  Data Store Write1 : DataStoreWrite  DataStoreName=RED_Rz_Elbow
  Data Store Write2 : DataStoreWrite  DataStoreName=RED_Rz_Wrist
  Data Store Write3 : DataStoreWrite  DataStoreName=RED_RzD_Shoulder
  Data Store Write4 : DataStoreWrite  DataStoreName=RED_RzD_Elbow
  Data Store Write5 : DataStoreWrite  DataStoreName=RED_RzD_Wrist
  Read Joint Positions using Dynamixel Encoders : MainLibrary/Dynamixel Functions/Read Joint Positions using  Dynamixel Encoders  SampleTime=baseRate
      settings: SourceProductName=SPOT Custom Library
  wires:
  Read Joint Positions using Dynamixel Encoders/1 -> Correct for dropouts/1(In1)
  Correct for dropouts/1(FixedInput) -> Data Store Write/1
  Read Joint Positions using Dynamixel Encoders/2 -> Correct for dropouts1/1(In1)
  Correct for dropouts1/1(FixedInput) -> Data Store Write1/1
  Correct for dropouts2/1(FixedInput) -> Data Store Write2/1
  Read Joint Positions using Dynamixel Encoders/3 -> Correct for dropouts2/1(In1)
  Read Joint Positions using Dynamixel Encoders/4 -> Data Store Write3/1
  Read Joint Positions using Dynamixel Encoders/5 -> Data Store Write4/1
  Read Joint Positions using Dynamixel Encoders/6 -> Data Store Write5/1
